simulink model "ME322_Exercise_2_Simulink - Copy"  (R2024b)
settings: Solver=VariableStepAuto  StartTime=0.0  StopTime=10.0  RelTol=1e-6
undefined symbols (not defined in the file): A, b_s, b_t, k_s, k_t, lambda, m_c, m_u, x_dot_c
settings Model: Creator=caidenbonney  LastModifiedBy=Caide

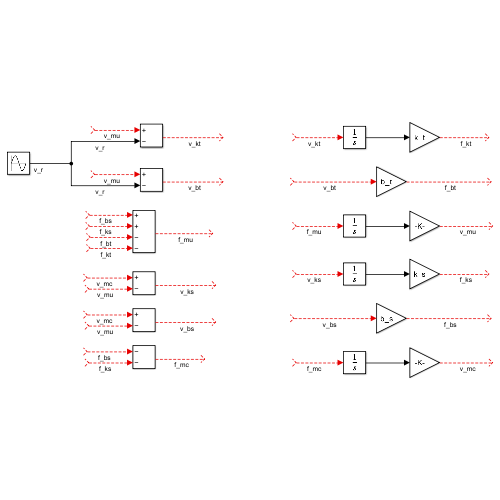
[thumbnail: Simulink's stored preview of the top-level diagram]
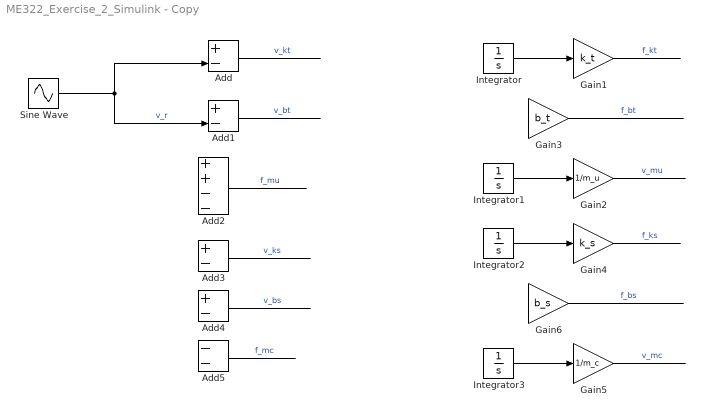
== system ME322_Exercise_2_Simulink - Copy ==
  Add{,1,3..4} (4 alike) : Sum  Inputs=+-
  Add2 : Sum  Inputs=++--
  Add5 : Sum  Inputs=--
  Gain1 : Gain  Gain=k_t
  Gain2 : Gain  Gain=1/m_u
  Gain3 : Gain  Gain=b_t
  Gain4 : Gain  Gain=k_s
  Gain5 : Gain  Gain=1/m_c
  Gain6 : Gain  Gain=b_s
  Integrator{,1..3} (4 alike) : Integrator
  Sine Wave : Sin  Amplitude=(2*pi*A*x_dot_c)/lambda  Frequency=(2*pi*x_dot_c)/lambda  SampleTime=0
  wires:
  ? -> Integrator/1  "v_kt"
  Integrator/1 -> Gain1/1
  Gain1/1 -> ?  "f_kt"
  Gain3/1 -> ?  "f_bt"
  ? -> Gain3/1  "v_bt"
  Gain2/1 -> ?  "v_mu"
  Integrator1/1 -> Gain2/1
  ? -> Integrator1/1  "f_mu"
  ? -> Integrator3/1  "f_mc"
  Integrator3/1 -> Gain5/1
  Gain5/1 -> ?  "v_mc"
  ? -> Gain6/1  "v_bs"
  Gain6/1 -> ?  "f_bs"
  Gain4/1 -> ?  "f_ks"
  Integrator2/1 -> Gain4/1
  ? -> Integrator2/1  "v_ks"
  ? -> Add/1  "v_mu"
  Add/1 -> ?  "v_kt"
  Add1/1 -> ?  "v_bt"
  ? -> Add1/1  "v_mu"
  ? -> Add2/1  "f_bs"
  ? -> Add2/2  "f_ks"
  ? -> Add2/3  "f_bt"
  ? -> Add2/4  "f_kt"
  Add2/1 -> ?  "f_mu"
  ? -> Add3/1  "v_mc"
  ? -> Add3/2  "v_mu"
  Add3/1 -> ?  "v_ks"
  Add4/1 -> ?  "v_bs"
  ? -> Add4/2  "v_mu"
  ? -> Add4/1  "v_mc"
  ? -> Add5/1  "f_bs"
  ? -> Add5/2  "f_ks"
  Add5/1 -> ?  "f_mc"
  Sine Wave/1 -> Add/2, Add1/2  "v_r"
